simulink model "sf_path"  (R2023b)
settings: Solver=VariableStepAuto  StartTime=0.0  StopTime=10.0  RelTol=1e-3
libraries: simulink x1
settings Model: Creator=fsp  LastModifiedBy=fsp

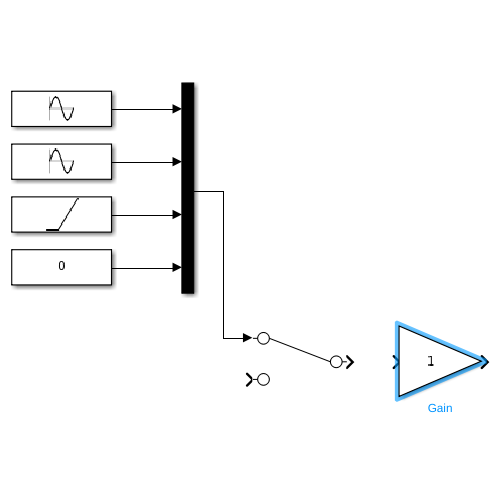
[thumbnail: Simulink's stored preview of the top-level diagram]
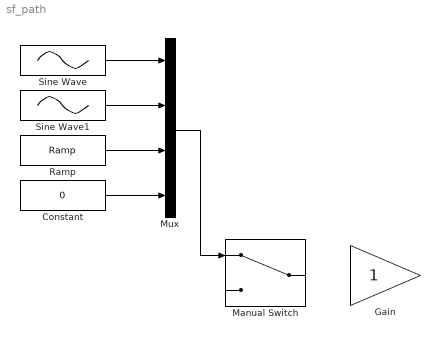
== system sf_path ==
  Constant : Constant  Value=0
  Gain : Gain
  Manual Switch : ManualSwitch
  Mux : Mux
  Ramp : simulink/Sources/Ramp  slope=1  start=0  InitialOutput=0
  Sine Wave : Sin  SampleTime=0
  Sine Wave1 : Sin  SampleTime=0
  wires:
  Sine Wave/1 -> Mux/1
  Sine Wave1/1 -> Mux/2
  Ramp/1 -> Mux/3
  Constant/1 -> Mux/4
  Mux/1 -> Manual Switch/1
